simulink model "LQR_DW"  (R2022b)
settings: Solver=FixedStepAuto  StartTime=0.0  StopTime=5  FixedStep=0.01  RelTol=1e-3
values from neighbouring files (symbols this model uses):
  B = [ ... (first row only)    [KF.m]    (also in Luenberger.m = [0)
  K = P_pre * H' * inv(H * P_pre * H' + R)    [KF.m]
undefined symbols (not defined in the file or in its folder): A, C, D, SP, threshold
libraries: simulink x1, eeLuenbergerObserver x1
settings Model: Creator=miakho  LastModifiedBy=miakho

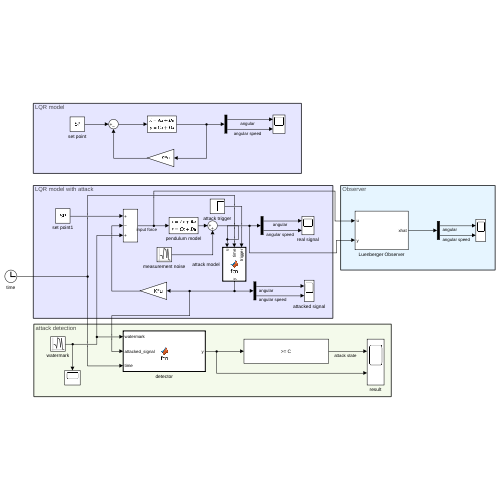
[thumbnail: Simulink's stored preview of the top-level diagram]
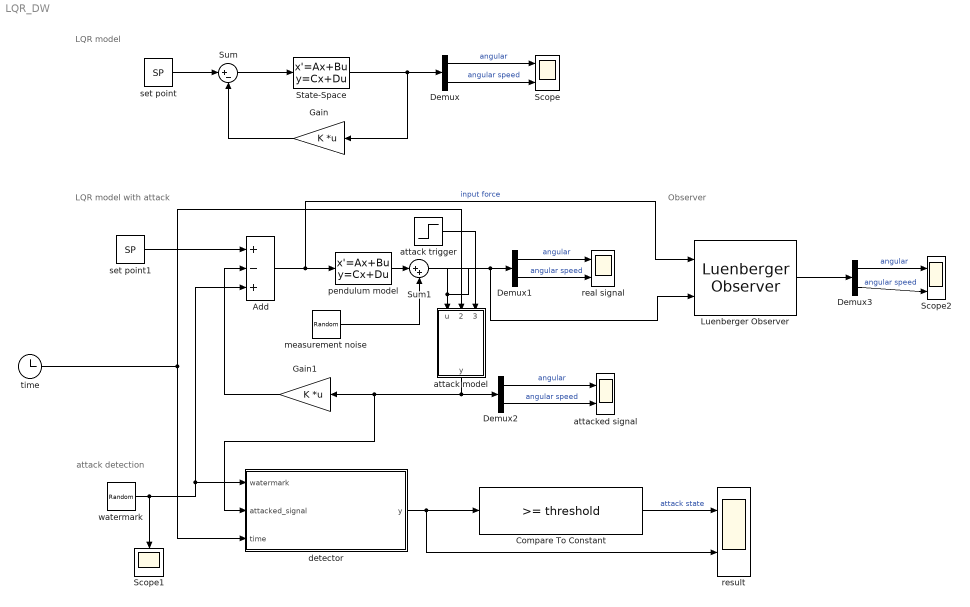
== system LQR_DW ==
  note: Observer
  note: attack detection
  note: LQR model
  note: LQR model with attack
  Add : Sum  Inputs=+-+
  Compare To Constant : simulink/Logic and Bit Operations/Compare To Constant  relop=>=  const=threshold  OutDataTypeStr=boolean
  Demux{,1..3} (4 alike) : Demux  Outputs=2
  Gain : Gain  Gain=K  Multiplication=Matrix(K*u)
  Gain1 : Gain  Gain=K  Multiplication=Matrix(K*u)
  Luenberger Observer : eeLuenbergerObserver/Luenberger Observer  StateSpaceType=Continuous-time  Ad=A  Bd=B  Cd=C  Dd=D  A=A  B=B  C=C  D=D  ObserverDesign=Desired eigenvalues  Ld=1  DesiredEigenvalues=[-20;-20]  x0=[0; 0]  Tsd=0.01  Ts=-1
      settings: LibrarySourceBlock=ee_sl_lib/Observers/Luenberger Observer
  Scope : Scope  NumInputPorts=2
  Scope1 : Scope
  Scope2 : Scope  NumInputPorts=2
  State-Space : StateSpace  A=A  B=B  C=C  D=D  InitialCondition=[5 0]  ParameterTunability=Unconstrained
  Sum : Sum  Inputs=|+-
  Sum1 : Sum  Inputs=|++
  attack model : MATLAB Function  TreatAsAtomicUnit=on
  attack trigger : Step  SampleTime=0
  attacked signal : Scope  NumInputPorts=2
  detector : MATLAB Function  TreatAsAtomicUnit=on
  measurement noise : RandomNumber  Variance=0.002  Seed=5  SampleTime=0.01
  pendulum model : StateSpace  A=A  B=B  C=C  D=D  InitialCondition=[5 0]  ParameterTunability=Unconstrained
  real signal : Scope  NumInputPorts=2
  result : Scope  NumInputPorts=2
  set point : Constant  Value=SP
  set point1 : Constant  Value=SP
  time : Clock
  watermark : RandomNumber  Variance=0.01  Seed=1  SampleTime=0.01
  wires:
  State-Space/1 -> Demux/1, Gain/1
  Demux/1 -> Scope/1  "angular"
  Demux/2 -> Scope/2  "angular speed"
  set point/1 -> Sum/1
  Sum/1 -> State-Space/1
  Gain/1 -> Sum/2
  Gain1/1 -> Add/2
  Add/1 -> Luenberger Observer/1, pendulum model/1  "input force"
  set point1/1 -> Add/1
  Demux1/2 -> real signal/2  "angular speed"
  Demux1/1 -> real signal/1  "angular"
  Sum1/1 -> Luenberger Observer/2, Demux1/1, attack model/1(u)
  attack model/1(y) -> Demux2/1, detector/2(attacked_signal), Gain1/1
  attack trigger/1 -> attack model/3(trigger)
  Demux2/1 -> attacked signal/1  "angular"
  Demux2/2 -> attacked signal/2  "angular speed"
  watermark/1 -> Add/3, detector/1(watermark), Scope1/1
  Compare To Constant/1 -> result/1  "attack state"
  detector/1(y) -> Compare To Constant/1, result/2
  time/1 -> attack model/2(time), detector/3(time)
  Luenberger Observer/1 -> Demux3/1
  Demux3/1 -> Scope2/1  "angular"
  Demux3/2 -> Scope2/2  "angular speed"
  pendulum model/1 -> Sum1/1
  measurement noise/1 -> Sum1/2

== matlab function LQR_DW/attack model ==
  settings: updateMethod=DISCRETE
  data: u input; time input; y output; trigger input
function y = fcn(u, time, trigger)
% input is the true value and the output is the attacked value'
% the step of the system
fixed_step = 0.01;
current_step = time/fixed_step+1;

% recieve and store the data of the input
persistent d_input;
if isempty(d_input)
    d_input=zeros(2,501);
else
    d_input(:,int32(current_step))=u;
end

% remember the last timestep
persistent replay_attack_accord;
if isempty(replay_attack_accord)
    replay_attack_accord=int32(0);
else
    if trigger==0
        replay_attack_accord=int32(current_step);
    end
end



%% choose attack type
% 0 is no attack, 1 is replay attack, 2 is Dos attack
attack_type = 1;

% no attack 
if attack_type==0
    y=u;
end

% replay attack
if attack_type==1
    if trigger==0
        y=u;
    else
        y=d_input(:,mod(int32(current_step)-replay_attack_accord,replay_attack_accord)+1);
    end
end

% Dos attack
if attack_type==2
    if trigger==0
        y = u;
    else
        y = u-u;
    end
end

end

== matlab function LQR_DW/detector ==
  settings: updateMethod=DISCRETE
  data: watermark input; y output; attacked_signal input; time input
function y = fcn(watermark, attacked_signal, time)

% the step of the system
fixed_step = 0.01;
current_step = time/fixed_step+1;
total_step = 501; %the step of the simulation

persistent d_watermark;
persistent d_attacked_signal;

if isempty(d_watermark)
    d_watermark=zeros(1,501);
    d_attacked_signal=zeros(2,501);
end

d_watermark(int32(current_step))=watermark;
d_attacked_signal(:,int32(current_step))=attacked_signal;

sum = 0.00000;
for i=1:int32(current_step)
    sum = sum + d_watermark(i);
end

mean = sum/current_step;

y = mean;
